simulink model "Mainframe"  (R2021a)
settings: Solver=FixedStepAuto  StartTime=0.0  StopTime=60  FixedStep=0.001  RelTol=1e-3
values from neighbouring files (symbols this model uses):
  den_lpf_d = den_lpf20    [Mainframe_init.m]    (also in load_autopilot.m)
  Emulated_FCC_IO_Delay = 7    [Mainframe_init.m]
  Enable_Gyros = 0    [Mainframe_init.m]
  Enable_INS = 0    [Mainframe_init.m]
  num_lpf_d = num_lpf20    [Mainframe_init.m]    (also in load_autopilot.m)
undefined symbols (not defined in the file or in its folder): act_dmp, act_omega, Actuator, Aerodynamics, aMode, Autopilot, AUX, c_b_WGS, c_be, c_flat, c_grav, c_h_geop0, c_h_geope, c_pa0, c_pe, c_r0, c_rot, c_rsma, c_Tmp0, d_siB_0, d_siB_max, d_siB_min, dd_siB_max, dd_siB_min, dev, DiscIntNeverNeededParam, e_pa, e_Tmp, fin_maxrate, flag_I_act_switch, flag_I_aero_switch, flag_I_flat, flag_I_gravity_switch, flag_I_rot, hcr, HIL_Data, JMMM_0, JMMM_e, JSPB_e, lat_0, lon_0, Mass_Props, mB_0, mM_0, mM_e, National_Instruments, Newton, pBII_0, PCIe, pMPB, pNPB, propellant_kg, prp_FBPB, prp_mdot, prp_T, pSPB, pwm_output1, qEG_0, qIB_0, qIE_0 ... (+31)
libraries: simulink_extras x38, simulink x31, custom_blocks x11, sldrtlib x10, aerolibcommonsys x4, px4Sensorslib x3, px4lib x3, aerolibnav x1
(part 5 of 17)

== system Mainframe/Non-linear Flight Dynamic Model/GRM_Airframe/weight_and_balance/center_of_gravity ==
  mB : Inport
  mM : Inport  Port=2
  1-D Lookup Table : Lookup_n-D  NumberOfTableDimensions=1  BreakpointsForDimension1=Mass_Props.propellant_bkpts  Table=Mass_Props.CGx_m_tbl  ExtrapMethod=Clip  UseLastTableValue=on  InternalRulePriority=Speed  RndMeth=Simplest  InputSameDT=on
      settings: AttributesFormatString=|
      | %<Table>
      | %<BreakpointsForDimension1>
  1-D Lookup Table3 : Lookup_n-D  NumberOfTableDimensions=1  BreakpointsForDimension1=Mass_Props.propellant_bkpts  Table=Mass_Props.CGy_m_tbl  ExtrapMethod=Clip  UseLastTableValue=on  InternalRulePriority=Speed  RndMeth=Simplest  InputSameDT=on
      settings: AttributesFormatString=|
      | %<Table>
      | %<BreakpointsForDimension1>
  1-D Lookup Table6 : Lookup_n-D  NumberOfTableDimensions=1  BreakpointsForDimension1=Mass_Props.propellant_bkpts  Table=Mass_Props.CGz_m_tbl  ExtrapMethod=Clip  UseLastTableValue=on  InternalRulePriority=Speed  RndMeth=Simplest  InputSameDT=on
      settings: AttributesFormatString=|
      | %<Table>
      | %<BreakpointsForDimension1>
  Add6 : Sum
  Add7 : Sum
  Add8 : Sum
  Constant10 : Constant  Value=unc_cg_x
  Constant11 : Constant  Value=unc_cg_y
  Constant12 : Constant  Value=unc_cg_z
  Terminator1 : Terminator
  Vector Concatenate1 : Concatenate  NumInputs=3
  mM D2 : InportShadow  Port=2
  mM D3 : InportShadow  Port=2
  pBPB : Outport  VectorParamsAs1DForOutWhenUnconnected=off
  wires:
  1-D Lookup Table6/1 -> Add8/1
  1-D Lookup Table3/1 -> Add7/1
  Vector Concatenate1/1 -> pBPB/1  "pBPB"
  1-D Lookup Table/1 -> Add6/1
  mM/1 -> 1-D Lookup Table/1
  mM D2/1 -> 1-D Lookup Table3/1
  mM D3/1 -> 1-D Lookup Table6/1
  Add6/1 -> Vector Concatenate1/1
  Constant10/1 -> Add6/2
  Constant11/1 -> Add7/2
  Add7/1 -> Vector Concatenate1/2
  Constant12/1 -> Add8/2
  Add8/1 -> Vector Concatenate1/3
  mB/1 -> Terminator1/1

== system Mainframe/Non-linear Flight Dynamic Model/GRM_Airframe/weight_and_balance/mass ==
  sim_time_launch : Inport
  1-D Lookup Table2 : Lookup_n-D  NumberOfTableDimensions=1  BreakpointsForDimension1=prp_T  Table=prp_mdot  ExtrapMethod=Clip  DiagnosticForOutOfRangeInput=Warning  UseLastTableValue=on  InternalRulePriority=Speed  RndMeth=Simplest  InputSameDT=on
  Constant : Constant  Value=0
  Constant1 : Constant  Value=mB_0
  Constant2 : Constant  Value=propellant_kg
      settings: AttributesFormatString=%<Value>
  Gain : Gain  Gain=-1
  Integrator1 : Integrator  InitialConditionSource=external
  Saturation : Saturate  UpperLimit=prp_T(end)  LowerLimit=0
      settings: AttributesFormatString=|
      | %<UpperLimit>
      | %<LowerLimit>
  Subtract1 : Sum
  Switch : Switch  Criteria=u2 > Threshold
  Switch1 : Switch  Criteria=u2 > Threshold
  mB_c : Outport  VectorParamsAs1DForOutWhenUnconnected=off
  mM : Outport  Port=2  VectorParamsAs1DForOutWhenUnconnected=off
  wires:
  Constant1/1 -> Subtract1/1
  Subtract1/1 -> mB_c/1  "mB_c"
  Switch/1 -> Switch1/2, Switch1/3, Saturation/1
  Constant/1 -> Switch/3
  sim_time_launch/1 -> Switch/1, Switch/2
  Saturation/1 -> 1-D Lookup Table2/1
  Switch1/1 -> mM/1, Subtract1/2  "mM"
  Constant2/1 -> Integrator1/2
  1-D Lookup Table2/1 -> Gain/1  "mdot_kgps"
  Gain/1 -> Integrator1/1
  Integrator1/1 -> Switch1/1  "propellant_remaining_kg"

== system Mainframe/Non-linear Flight Dynamic Model/GRM_Airframe/weight_and_balance/mass_uncertainty ==
  mB_c : Inport
  Add : Sum
  Constant : Constant  Value=unc_mB_bl
  Constant1 : Constant  Value=unc_mB_scale
  Product : Product
  mB : Outport  VectorParamsAs1DForOutWhenUnconnected=off
  wires:
  Constant/1 -> Add/1
  mB_c/1 -> Product/1
  Add/1 -> mB/1  "mB"
  Constant1/1 -> Product/2
  Product/1 -> Add/2

== system Mainframe/Non-linear Flight Dynamic Model/GRM_Airframe/weight_and_balance/moi ==
  pBPB : Inport
  mM : Inport  Port=2
  1-D Lookup Table : Lookup_n-D  NumberOfTableDimensions=1  BreakpointsForDimension1=Mass_Props.propellant_bkpts  Table=Mass_Props.Ixx_tbl  ExtrapMethod=Clip  UseLastTableValue=on  InternalRulePriority=Speed  RndMeth=Simplest  InputSameDT=on
      settings: AttributesFormatString=|
      | %<Table>
      | %<BreakpointsForDimension1>
  1-D Lookup Table1 : Lookup_n-D  NumberOfTableDimensions=1  BreakpointsForDimension1=Mass_Props.propellant_bkpts  Table=Mass_Props.Ixy_tbl  ExtrapMethod=Clip  UseLastTableValue=on  InternalRulePriority=Speed  RndMeth=Simplest  InputSameDT=on
      settings: AttributesFormatString=|
      | %<Table>
      | %<BreakpointsForDimension1>
  1-D Lookup Table2 : Lookup_n-D  NumberOfTableDimensions=1  BreakpointsForDimension1=Mass_Props.propellant_bkpts  Table=Mass_Props.Ixz_tbl  ExtrapMethod=Clip  UseLastTableValue=on  InternalRulePriority=Speed  RndMeth=Simplest  InputSameDT=on
      settings: AttributesFormatString=|
      | %<Table>
      | %<BreakpointsForDimension1>
  1-D Lookup Table3 : Lookup_n-D  NumberOfTableDimensions=1  BreakpointsForDimension1=Mass_Props.propellant_bkpts  Table=Mass_Props.Iyx_tbl  ExtrapMethod=Clip  UseLastTableValue=on  InternalRulePriority=Speed  RndMeth=Simplest  InputSameDT=on
      settings: AttributesFormatString=|
      | %<Table>
      | %<BreakpointsForDimension1>
  1-D Lookup Table4 : Lookup_n-D  NumberOfTableDimensions=1  BreakpointsForDimension1=Mass_Props.propellant_bkpts  Table=Mass_Props.Iyy_tbl  ExtrapMethod=Clip  UseLastTableValue=on  InternalRulePriority=Speed  RndMeth=Simplest  InputSameDT=on
      settings: AttributesFormatString=|
      | %<Table>
      | %<BreakpointsForDimension1>
  1-D Lookup Table5 : Lookup_n-D  NumberOfTableDimensions=1  BreakpointsForDimension1=Mass_Props.propellant_bkpts  Table=Mass_Props.Iyz_tbl  ExtrapMethod=Clip  UseLastTableValue=on  InternalRulePriority=Speed  RndMeth=Simplest  InputSameDT=on
      settings: AttributesFormatString=|
      | %<Table>
      | %<BreakpointsForDimension1>
  1-D Lookup Table6 : Lookup_n-D  NumberOfTableDimensions=1  BreakpointsForDimension1=Mass_Props.propellant_bkpts  Table=Mass_Props.Izx_tbl  ExtrapMethod=Clip  UseLastTableValue=on  InternalRulePriority=Speed  RndMeth=Simplest  InputSameDT=on
      settings: AttributesFormatString=|
      | %<Table>
      | %<BreakpointsForDimension1>
  1-D Lookup Table7 : Lookup_n-D  NumberOfTableDimensions=1  BreakpointsForDimension1=Mass_Props.propellant_bkpts  Table=Mass_Props.Izy_tbl  ExtrapMethod=Clip  UseLastTableValue=on  InternalRulePriority=Speed  RndMeth=Simplest  InputSameDT=on
      settings: AttributesFormatString=|
      | %<Table>
      | %<BreakpointsForDimension1>
  1-D Lookup Table8 : Lookup_n-D  NumberOfTableDimensions=1  BreakpointsForDimension1=Mass_Props.propellant_bkpts  Table=Mass_Props.Izz_tbl  ExtrapMethod=Clip  UseLastTableValue=on  InternalRulePriority=Speed  RndMeth=Simplest  InputSameDT=on
      settings: AttributesFormatString=|
      | %<Table>
      | %<BreakpointsForDimension1>
  Add : Sum  Commented=on
  Add4 : Sum  Commented=on
  Add5 : Sum  Commented=on
  Constant15 : Constant  Commented=on  Value=JSPB_e
  JMMM_linear_interpolation : Subsystem  Commented=on
  Matrix Concatenate : Concatenate  NumInputs=3  Mode=Multidimensional array  ConcatenateDimension=2
  Terminator : Terminator  Commented=on
  Vector Concatenate : Concatenate  NumInputs=3
  Vector Concatenate1 : Concatenate  NumInputs=3
  Vector Concatenate2 : Concatenate  NumInputs=3
  mM D{1..9} (9 alike) : InportShadow  Port=2
  moi_coordinate_transformation : Subsystem  Commented=on
  moi_uncertainty : Subsystem
  steiners_theorem_missile : Subsystem  Commented=on
  steiners_theorem_motor : Subsystem  Commented=on
  JBBB : Outport  VectorParamsAs1DForOutWhenUnconnected=off
  wires:
  mM/1 -> steiners_theorem_motor/2(mM), JMMM_linear_interpolation/1(mM)
  JMMM_linear_interpolation/1(JMMM) -> moi_coordinate_transformation/1(JMMM)
  moi_coordinate_transformation/1(JMMB) -> Add/2
  pBPB/1 -> steiners_theorem_missile/1(pBPB), steiners_theorem_motor/1(pBPB)
  steiners_theorem_motor/1(JM_deviation) -> Add/1
  Add/1 -> Add4/2  "JMBB"
  Constant15/1 -> Add5/1
  Add5/1 -> Add4/1  "JSBB"
  steiners_theorem_missile/1(J_deviation) -> Add5/2
  Add4/1 -> Terminator/1  "JBBB_c"
  moi_uncertainty/1(JBBB) -> JBBB/1
  mM D1/1 -> 1-D Lookup Table/1
  mM D2/1 -> 1-D Lookup Table3/1
  mM D3/1 -> 1-D Lookup Table6/1
  mM D4/1 -> 1-D Lookup Table1/1
  mM D5/1 -> 1-D Lookup Table4/1
  mM D6/1 -> 1-D Lookup Table7/1
  mM D7/1 -> 1-D Lookup Table2/1
  mM D8/1 -> 1-D Lookup Table5/1
  mM D9/1 -> 1-D Lookup Table8/1
  1-D Lookup Table6/1 -> Vector Concatenate/3
  1-D Lookup Table3/1 -> Vector Concatenate/2
  1-D Lookup Table/1 -> Vector Concatenate/1
  1-D Lookup Table1/1 -> Vector Concatenate1/1
  1-D Lookup Table4/1 -> Vector Concatenate1/2
  1-D Lookup Table7/1 -> Vector Concatenate1/3
  1-D Lookup Table2/1 -> Vector Concatenate2/1
  1-D Lookup Table5/1 -> Vector Concatenate2/2
  1-D Lookup Table8/1 -> Vector Concatenate2/3
  Vector Concatenate/1 -> [MOI_matrix_col1]
  Vector Concatenate1/1 -> [MOI_matrix_col2]
  Vector Concatenate2/1 -> [MOI_matrix_col3]
  [MOI_matrix_col1] -> Matrix Concatenate/1
  [MOI_matrix_col2] -> Matrix Concatenate/2
  [MOI_matrix_col3] -> Matrix Concatenate/3
  Matrix Concatenate/1 -> moi_uncertainty/1(JBBB_c)  "JBBB_c"

== system Mainframe/Non-linear Flight Dynamic Model/Subsystem1/Extract States/Assemble_States_Bus1 ==
  Translation_States : Inport
  Rotation_States : Inport  Port=2
  Translation_States_Dot : Inport  Port=3
  Rotation_States_Dot : Inport  Port=4
  Attitude_States : Inport  Port=5
  POS_NED : Inport  Port=6
  POS_NED_dot : Inport  Port=7
  Bus Creator{1,4..6,8,12..13} (7 alike) : BusCreator  Inputs=3
  Bus Creator3 : BusCreator  Inputs=7
  Bus Creator7 : BusCreator  Inputs=2
  Bus Creator9 : BusCreator  Inputs=4
  Demux : Demux
  Demux{1..7} (7 alike) : Demux  Outputs=3
  Rotation Angles to Quaternions : Subsystem  mask(Ang2Quat){rotationOrder=ZYX, aMode=aMode}
      mask prompts: rotationOrder "shared_aeroblks:sharedaeroblktransform:blockAng2QuatParamRotationOrder"
      mask help: shared_aeroblks:sharedaeroblktransform:blockAng2QuatDesc
      mask init:
      | if aerosharedtest(gcb)
      |     ports=aerosharedicon('sharedang2quat');
      | else
      |     ports=sharedautoicon('sharedang2quat');
      | end
      settings: AttributesFormatString=Rotation Order: %<rotationOrder>
      mask Help: eval('if license(''test'',''Aerospace_Blockset'')aerosharedhelp(''rotation_angles_to_quaternions'');elseif license(''test'',''Powertrain_Blockset'')sharedautohelp(''rotation_angles_to_quaternions'');end')
      mask TypeOptions rotationOrder: shared_aeroblks:sharedaeroblktransform:blockParamComboZYX | shared_aeroblks:sharedaeroblktransform:blockParamComboZYZ | shared_aeroblks:sharedaeroblktransform:blockParamComboZXY | shared_aeroblks:sharedaeroblktransform:blockParamComboZXZ | shared_aeroblks:sharedaeroblktransform:blockParamComboYXZ | shared_aeroblks:sharedaeroblktransform:blockParamComboYXY | shared_aeroblks:sharedaeroblktransform:blockParamComboYZX | shared_aeroblks:sharedaeroblktransform:blockParamComboYZY | shared_aeroblks:sharedaeroblktransform:blockParamComboXYZ | shared_aeroblks:sharedaeroblktransform:blockParamComboXYX | shared_aeroblks:sharedaeroblktransform:blockParamComboXZY | shared_aeroblks:sharedaeroblktransform:blockParamComboXZX
      mask DialogControl rotationOrder Prompt: Rotation order:
      mask Display:
      | port_label('input',1,'[R_1,R_2,R_3]','texmode','on')
      | port_label('output',1,'q','texmode','on')
  Selector : Selector  InputPortWidth=3  IndexOptions=Index vector (dialog)  Indices=[3,2,1]  OutputSizes=1
  Three-axis Inertial Measurement Unit3 : Subsystem  Commented=on  mask(Three-axis Inertial Measurement Unit){units=Metric (MKS), imu=[0 0 0], i_Ts=0, dtype_a=on, w_a=190, z_a=0.707, a_sf_cc=[1 0 0; 0 1 0; 0 0 1], a_bias=[0 0 0], a_sat=[-inf  -inf  -inf  inf inf inf], dtype_g=on, w_g=190, z_g=0.707, g_sf_cc=[1 0 0; 0 1 0; 0 0 1], g_bias=[0 0 0], g_sens=[0 0 0], g_sat=[-inf  -inf  -inf  inf inf inf], i_rand=on, i_seeds=[23093 23094 23095 23096 23097 23098], i_pow=[0.001 0.001 0.001 0.0001 0.0001 0.0001]}
      mask prompts: units "aeroblks:aeroblknav:blockThreeaxisInertialMeasurementUnitParamUnits"; imu "aeroblks:aeroblknav:blockThreeaxisInertialMeasurementUnitParamIMUlocation"; i_Ts "aeroblks:aeroblknav:blockThreeaxisInertialMeasurementUnitParamUpdaterate"; dtype_a "aeroblks:aeroblknav:blockThreeaxisInertialMeasurementUnitParamSecondorderdynamicsforaccelerometer"; w_a "aeroblks:aeroblknav:blockThreeaxisInertialMeasurementUnitParamAccelerometernaturalfrequencyradsec"; z_a "aeroblks:aeroblknav:blockThreeaxisInertialMeasurementUnitParamAccelerometerdampingratio"; a_sf_cc "aeroblks:aeroblknav:blockThreeaxisInertialMeasurementUnitParamAccelerometerscalefactorandcrosscoupling"; a_bias "aeroblks:aeroblknav:blockThreeaxisInertialMeasurementUnitParamAccelerometermeasurementbias"; a_sat "aeroblks:aeroblknav:blockThreeaxisInertialMeasurementUnitParamAccelerometerupperandlowerlimits"; dtype_g "aeroblks:aeroblknav:blockThreeaxisInertialMeasurementUnitParamSecondorderdynamicsforgyro"; w_g "aeroblks:aeroblknav:blockThreeaxisInertialMeasurementUnitParamGyronaturalfrequencyradsec"; z_g "aeroblks:aeroblknav:blockThreeaxisInertialMeasurementUnitParamGyrodampingratio"; g_sf_cc "aeroblks:aeroblknav:blockThreeaxisInertialMeasurementUnitParamGyroscalefactorsandcrosscoupling"; g_bias "aeroblks:aeroblknav:blockThreeaxisInertialMeasurementUnitParamGyromeasurementbias"; g_sens "aeroblks:aeroblknav:blockThreeaxisInertialMeasurementUnitParamGsensitivebias"; g_sat "aeroblks:aeroblknav:blockThreeaxisInertialMeasurementUnitParamGyroupperandlowerlimits"; i_rand "aeroblks:aeroblknav:blockThreeaxisInertialMeasurementUnitParamNoiseon"; i_seeds "aeroblks:aeroblknav:blockThreeaxisInertialMeasurementUnitParamNoiseseeds"; i_pow "aeroblks:aeroblknav:blockThreeaxisInertialMeasurementUnitParamNoisepower"
      mask help: aeroblks:aeroblknav:blockThreeaxisInertialMeasurementUnitDesc
      mask init:
      | block = gcb;   
      | ports=aeroicon('aeroblkimu','icon');
      mask Help: eval('asbhelp');
      mask TypeOptions units: aeroblks:aeroblknav:blockThreeaxisInertialMeasurementUnitParamComboMetricMKS | aeroblks:aeroblknav:blockThreeaxisInertialMeasurementUnitParamComboEnglish
      mask Callback dtype_a: aeroicon('aeroblkimu')
      mask Callback dtype_g: aeroicon('aeroblkimu')
      mask Callback i_rand: aeroicon('aeroblkimu')
      mask DialogControl ParameterTabVar0 Prompt: Main
      mask DialogControl units Prompt: Units:
      mask DialogControl imu Prompt: IMU location:
      mask DialogControl i_Ts Prompt: Update rate:
      mask DialogControl ParameterTabVar01 Prompt: Accelerometer
      mask DialogControl dtype_a Prompt: Second-order dynamics for accelerometer
      mask DialogControl w_a Prompt: Accelerometer natural frequency (rad/sec):
      mask DialogControl z_a Prompt: Accelerometer damping ratio:
      mask DialogControl a_sf_cc Prompt: Accelerometer scale factor and cross-coupling:
      mask DialogControl a_bias Prompt: Accelerometer measurement bias:
      mask DialogControl a_sat Prompt: Accelerometer upper and lower limits:
      mask DialogControl ParameterTabVar012 Prompt: Gyroscope
      mask DialogControl dtype_g Prompt: Second-order dynamics for gyro
      mask DialogControl w_g Prompt: Gyro natural frequency (rad/sec):
      mask DialogControl z_g Prompt: Gyro damping ratio:
      mask DialogControl g_sf_cc Prompt: Gyro scale factors and cross-coupling:
      mask DialogControl g_bias Prompt: Gyro measurement bias:
      mask DialogControl g_sens Prompt: G-sensitive bias:
      mask DialogControl g_sat Prompt: Gyro upper and lower limits:
      mask DialogControl ParameterTabVar0123 Prompt: Noise
      mask DialogControl i_rand Prompt: Noise on
      mask DialogControl i_seeds Prompt: Noise seeds:
      mask DialogControl i_pow Prompt: Noise power:
      mask Display:
      | port_label(ports(1).type,ports(1).port,ports(1).txt,'texmode','on');
      | port_label(ports(2).type,ports(2).port,ports(2).txt,'texmode','on');
      | port_label(ports(3).type,ports(3).port,ports(3).txt,'texmode','on');
      | port_label(ports(4).type,ports(4).port,ports(4).txt,'texmode','on');
      | port_label(ports(5).type,ports(5).port,ports(5).txt,'texmode','on');
      | port_label(ports(6).type,ports(6).port,ports(6).txt,'texmode','on');
      | port_label(ports(7).type,ports(7).port,ports(7).txt,'texmode','on');
  States : Outport  VectorParamsAs1DForOutWhenUnconnected=off
  wires:
  Bus Creator7/1 -> Bus Creator3/5  "Attitude_States"
  Demux/3 -> Bus Creator9/3  "quat_2"
  Demux/4 -> Bus Creator9/4  "quat_3"
  Demux/1 -> Bus Creator9/1  "quat_0"
  Bus Creator9/1 -> Bus Creator7/2  "ATT_Quaternions"
  Bus Creator12/1 -> Bus Creator3/6  "POS_NED"
  Demux/2 -> Bus Creator9/2  "quat_1"
  Bus Creator8/1 -> Bus Creator7/1  "ATT_Euler"
  Bus Creator4/1 -> Bus Creator3/1  "Translation_States"
  Bus Creator6/1 -> Bus Creator3/2  "Rotation_States"
  Bus Creator5/1 -> Bus Creator3/3  "Translation_States_Dot"
  Rotation Angles to Quaternions/1(Quat) -> Demux/1
  Demux6/3 -> Bus Creator12/3  "POS_z_NED_m"
  Demux6/2 -> Bus Creator12/2  "POS_y_NED_m"
  Demux6/1 -> Bus Creator12/1  "POS_x_NED_m"
  Demux5/3 -> Bus Creator8/3  "Psi_rad"
  Demux5/2 -> Bus Creator8/2  "Theta_rad"
  Demux5/1 -> Bus Creator8/1  "Phi_rad"
  Demux2/3 -> Bus Creator6/3  "r_radDs"
  Demux2/2 -> Bus Creator6/2  "q_radDs"
  Demux2/1 -> Bus Creator6/1  "p_radDs"
  Demux3/3 -> Bus Creator5/3  "w_dot_mDs2"
  Demux3/2 -> Bus Creator5/2  "v_dot_mDs2"
  Demux3/1 -> Bus Creator5/1  "u_dot_mDs2"
  Demux1/3 -> Bus Creator4/3  "w_mDs"
  Demux1/2 -> Bus Creator4/2  "v_mDs"
  Demux1/1 -> Bus Creator4/1  "u_mDs"
  Bus Creator13/1 -> Bus Creator3/4  "Rotation_States_Dot"
  Demux4/1 -> Bus Creator13/1  "p_dot_radDs2"
  Demux4/2 -> Bus Creator13/2  "q_dot_radDs2"
  Demux4/3 -> Bus Creator13/3  "r_dot_radDs2"
  Translation_States/1 -> Demux1/1
  Rotation_States/1 -> Demux2/1
  Translation_States_Dot/1 -> Demux3/1
  Rotation_States_Dot/1 -> Demux4/1
  Attitude_States/1 -> Selector/1, Demux5/1
  POS_NED/1 -> Demux6/1
  Bus Creator3/1 -> States/1  "FDM_States"
  Selector/1 -> Rotation Angles to Quaternions/1("R1, R2, R3")
  POS_NED_dot/1 -> Demux7/1
  Demux7/2 -> Bus Creator1/2  "POS_y_NED_dot_m"
  Demux7/3 -> Bus Creator1/3  "POS_z_NED_dot_m"
  Bus Creator1/1 -> Bus Creator3/7  "POS_NED_dot"
  Demux7/1 -> Bus Creator1/1  "POS_x_NED_dot_m"

== system Mainframe/Non-linear Flight Dynamic Model/Subsystem1/Extract States/quaternion_to_euler_angles1 ==
  note: Um numerische Probleme zu
      | vermeiden, wird hier eine Saturiierung
      | benutzt.
  note: Outputs [size]:
      |
      | roll angle [1]
      | pitch angle [1]
      | yaw angle [1]
  note: Inputs [size]:
      |
      | quaternion [4]
  q : Inport  PortDimensions=4
  Add : Sum
  Add1 : Sum  Inputs=+--
  Add2 : Sum  Inputs=+-
  Add3 : Sum
  Add4 : Sum  Inputs=+--
  Complex to Real-Imag : ComplexToRealImag  Output=Real
  Constant : Constant  Value=0.5
  Constant1 : Constant  Value=0.5
  Demux : Demux
  Gain : Gain  Gain=2
  Product{,1..9} (10 alike) : Product
  Saturation : Saturate  UpperLimit=1  LowerLimit=-1
      settings: AttributesFormatString=|
      | %<UpperLimit>
      | %<LowerLimit>
  Trigonometric Function : Trigonometry  Operator=atan2
  Trigonometric Function1 : Trigonometry  Operator=asin
  Trigonometric Function2 : Trigonometry  Operator=atan2
  Vector Concatenate : Concatenate  NumInputs=3
  eulx : Outport  VectorParamsAs1DForOutWhenUnconnected=off
  wires:
  Vector Concatenate/1 -> Complex to Real-Imag/1
  Complex to Real-Imag/1 -> eulx/1
  Trigonometric Function2/1 -> Vector Concatenate/3
  Trigonometric Function1/1 -> Vector Concatenate/2
  Trigonometric Function/1 -> Vector Concatenate/1
  Add/1 -> Trigonometric Function/1
  Product1/1 -> Add/2
  Product/1 -> Add/1
  Product3/1 -> Add1/3
  Product2/1 -> Add1/2
  Product5/1 -> Add2/2
  Product4/1 -> Add2/1
  Product7/1 -> Add3/2
  Product6/1 -> Add3/1
  Add3/1 -> Trigonometric Function2/1
  Add4/1 -> Trigonometric Function2/2
  Add2/1 -> Gain/1
  Add1/1 -> Trigonometric Function/2
  q/1 -> Demux/1
  Demux/4 -> Product7/2, Product4/2, Product/2  "4"
  Demux/1 -> Product2/2, Product2/1, Product/1, Product6/1, Product5/1  "1"
  Demux/2 -> Product4/1, Product3/2, Product3/1, Product1/1, Product8/2, Product8/1, Product6/2  "2"
  Constant/1 -> Add1/1
  Product9/1 -> Add4/3
  Product8/1 -> Add4/2
  Constant1/1 -> Add4/1
  Demux/3 -> Product9/2, Product9/1, Product7/1, Product1/2, Product5/2  "3"
  Gain/1 -> Saturation/1
  Saturation/1 -> Trigonometric Function1/1

== system Mainframe/Non-linear Flight Dynamic Model/Subsystem1/Fin Deflections/Degrees to Radians ==
  Degrees in : Inport
  Gain1 : Gain  Gain=pi/180  SaturateOnIntegerOverflow=on  OutDataTypeStr=Inherit: Same as input  ParamDataTypeStr=Inherit: Same as input
  Radians out : Outport  InitialOutput=0  VectorParamsAs1DForOutWhenUnconnected=off
  wires:
  Gain1/1 -> Radians out/1
  Degrees in/1 -> Gain1/1

== system Mainframe/Non-linear Flight Dynamic Model/Subsystem1/Fin Deflections/Degrees to Radians1 ==
  Degrees in : Inport
  Gain1 : Gain  Gain=pi/180  SaturateOnIntegerOverflow=on  OutDataTypeStr=Inherit: Same as input  ParamDataTypeStr=Inherit: Same as input
  Radians out : Outport  InitialOutput=0  VectorParamsAs1DForOutWhenUnconnected=off
  wires:
  Gain1/1 -> Radians out/1
  Degrees in/1 -> Gain1/1

== system Mainframe/Non-linear Flight Dynamic Model/Subsystem1/Fin Deflections/Degrees to Radians2 ==
  Degrees in : Inport
  Gain1 : Gain  Gain=pi/180  SaturateOnIntegerOverflow=on  OutDataTypeStr=Inherit: Same as input  ParamDataTypeStr=Inherit: Same as input
  Radians out : Outport  InitialOutput=0  VectorParamsAs1DForOutWhenUnconnected=off
  wires:
  Gain1/1 -> Radians out/1
  Degrees in/1 -> Gain1/1

== system Mainframe/Non-linear Flight Dynamic Model/Subsystem1/Fin Deflections/control_allocation ==
  fin_cmd : Inport
  Constant7 : Constant  Value=Tr4r3
  Product : Product  Multiplication=Matrix(*)
  siB_cmd : Outport  VectorParamsAs1DForOutWhenUnconnected=off
  wires:
  Product/1 -> siB_cmd/1  "siB_cmd"
  fin_cmd/1 -> Product/2
  Constant7/1 -> Product/1

== system Mainframe/Non-linear Flight Dynamic Model/Subsystem1/GRM_Airframe/aerodynamics ==
  str_flow : Inport
  fin : Inport  Port=2
  wab : Inport  Port=3
  env_glbl : Inport  Port=4
  Bus Selector : BusSelector  OutputSignals=qdynB,MaB,alB,beB,hBE,wBIB_star
  Bus Selector1 : BusSelector  OutputSignals=afinB
  Bus Selector2 : BusSelector  OutputSignals=pBPB
  aerodynamic_via_lookup : Subsystem
  logic_base_drag : Subsystem
  aero : Outport  VectorParamsAs1DForOutWhenUnconnected=off
  wires:
  str_flow/1 -> Bus Selector/1
  wab/1 -> Bus Selector2/1
  fin/1 -> Bus Selector1/1
  Bus Selector2/1 -> aerodynamic_via_lookup/1(pBPB)  "<pBPB>"
  Bus Selector/1 -> aerodynamic_via_lookup/2(qdynB)  "<qdynB>"
  Bus Selector/2 -> aerodynamic_via_lookup/3(MaB)  "<MaB>"
  Bus Selector/3 -> aerodynamic_via_lookup/4(alB)  "<alB>"
  Bus Selector/4 -> aerodynamic_via_lookup/5(beB)  "<beB>"
  Bus Selector/5 -> aerodynamic_via_lookup/6(hBE)  "<hBE>"
  Bus Selector1/1 -> aerodynamic_via_lookup/8(afinB)  "<afinB>"
  Bus Selector/6 -> aerodynamic_via_lookup/7(wBIB_star)  "<wBIB_star>"
  aerodynamic_via_lookup/1(aero_bus) -> aero/1
  env_glbl/1 -> logic_base_drag/1(env_glbl)
  logic_base_drag/1(flag_base_drag) -> aerodynamic_via_lookup/9(flag_I_prp)

== system Mainframe/Non-linear Flight Dynamic Model/Subsystem1/GRM_Airframe/environment ==
  flight_dyn : Inport
  env_glbl : Inport  Port=2
  Bus Creator1 : BusCreator  Inputs=2
  Bus Creator2 : BusCreator  Inputs=2
  Bus Selector : BusSelector  OutputSignals=lon,lat,hBE
  Bus Selector1 : BusSelector  OutputSignals=atm_dyn_bus
  Saturation : Saturate  UpperLimit=inf  LowerLimit=eps
      settings: AttributesFormatString=|
      | %<UpperLimit>
      | %<LowerLimit>
  WGS84_Gravitation : Subsystem  mask{flg_omega_enabled=on}
      mask prompts: flg_omega_enabled "Zentripetalbeschleunigung mitberechnen"
      mask help:
      | Dieser Block berechnet die Gravitation für das idealisierte WGS84
      | Ellipsoid. Die Berechnung ist hierbei nach dem Technical Report
      | "Department of Defense World Geodetic System 1984", NIMA TR8350.2,
      | Third Edition, Amendment 1 vom 3 Januar 2000 implementiert.
      | Das Modell ist gültig für alle Höhen über dem WGS84 Referenzellipsoid, und
      | ist somit der reinen Taylorexpansion des Somigliana Modells überlegen
      | (siehe Kapitel 4.3 des WGS84 reports).
      |
      | ---------------------------------------------------------------------------
      | Longitude [rad]: Nach WGS84 definierte Geodätische Länge.  (lambda)
      | Lattitude [rad]: Nach WGS84 definierte Geodätische Breite. (phi)
      | Height [m]: Höhe über dem WGS84 Referenzellipsoid.
      mask init:
      | [ c_rsma, c_b_WGS, c_grav, c_rot] = init_WGS84_Gravitationsmodell();
  atmosphere_static_ISO_2533 : Subsystem
  convert_to_local_frame : Subsystem
  env : Outport  VectorParamsAs1DForOutWhenUnconnected=off
  wires:
  convert_to_local_frame/1(gBG) -> Bus Creator2/1
  flight_dyn/1 -> Bus Selector/1
  WGS84_Gravitation/1(gE) -> convert_to_local_frame/1(gE)
  Bus Selector/1 -> WGS84_Gravitation/1(lon)  "<lon>"
  Bus Selector/3 -> atmosphere_static_ISO_2533/1(hBE), Saturation/1  "<hBE>"
  Bus Creator2/1 -> env/1  "env_bus"
  Bus Selector/2 -> WGS84_Gravitation/2(lat)  "<lat>"
  Bus Creator1/1 -> Bus Creator2/2  "atm_bus"
  Saturation/1 -> WGS84_Gravitation/3(h)
  atmosphere_static_ISO_2533/1(atm_stat) -> Bus Creator1/1  "atm_stat_bus"
  env_glbl/1 -> Bus Selector1/1, atmosphere_static_ISO_2533/2(env_glbl)
  Bus Selector1/1 -> Bus Creator1/2  "<atm_dyn_bus>"

== system Mainframe/Non-linear Flight Dynamic Model/Subsystem1/GRM_Airframe/fin_actuators ==
  cmd : Inport
  Bus Creator3 : BusCreator  Inputs=7
  Bus Selector : BusSelector  OutputSignals=siB_cmd
  Constant : Constant  Value=flag_I_act_switch
  Constant7 : Constant  Value=tRRR
  Demux : Demux
  Rudder : Subsystem  mask{siB_max=siB_max, siB_min=siB_min, d_siB_max=d_siB_max, d_siB_min=d_siB_min, dd_siB_max=dd_siB_max, dd_siB_min=dd_siB_min, omega=act_omega, dmp=act_dmp, unc_bl=unc_act_bl, unc_scale=unc_act_scale, unc_off=unc_act_off, siB_0=siB_0, d_siB_0=d_siB_0}
      mask prompts: siB_max "Obere Limitierung des Ruderstellwinkels in [rad]"; siB_min "Untere Limitierung des Ruderstellwinkels in [rad]"; d_siB_max "Obere Limitierung der Ruderstellwinkelgeschwindigkeit in [rad/s]"; d_siB_min "Untere Limitierung der Ruderstellwinkelgeschwindigkeit in [rad/s]"; dd_siB_max "Obere Limitierung der Ruderstellwinkelbeschleunigung in [rad/s^2]"; dd_siB_min "Untere Limitierung der Ruderstellwinkelbeschleunigung in [rad/s^2]"; omega "Eckfrequenz in [Hz]"; dmp "Dämpfung in [kg/s]"; unc_bl "Rückschlag des Aktuators (Backlash) in [rad]"; unc_scale "Skalenfehler in [-]"; unc_off "Versatz (Offset) in [rad]"; siB_0 "Startwert Ruderwinkel in [rad]"; d_siB_0 "Startwert Ruderwinkelgeschwindigkeiten in [rad/s]"
      mask DialogControl ParameterGroupVar Prompt: Limitierungen
      mask DialogControl Container3 Prompt: Dynamik
      mask DialogControl Container4 Prompt: Aktuatorfehler
      mask DialogControl Container5 Prompt: Startwerte
  Rudder1 : Subsystem  mask{siB_max=siB_max, siB_min=siB_min, d_siB_max=d_siB_max, d_siB_min=d_siB_min, dd_siB_max=dd_siB_max, dd_siB_min=dd_siB_min, omega=act_omega, dmp=act_dmp, unc_bl=unc_act_bl, unc_scale=unc_act_scale, unc_off=unc_act_off, siB_0=siB_0, d_siB_0=d_siB_0}
      mask prompts: siB_max "Obere Limitierung des Ruderstellwinkels in [rad]"; siB_min "Untere Limitierung des Ruderstellwinkels in [rad]"; d_siB_max "Obere Limitierung der Ruderstellwinkelgeschwindigkeit in [rad/s]"; d_siB_min "Untere Limitierung der Ruderstellwinkelgeschwindigkeit in [rad/s]"; dd_siB_max "Obere Limitierung der Ruderstellwinkelbeschleunigung in [rad/s^2]"; dd_siB_min "Untere Limitierung der Ruderstellwinkelbeschleunigung in [rad/s^2]"; omega "Eckfrequenz in [Hz]"; dmp "Dämpfung in [kg/s]"; unc_bl "Rückschlag des Aktuators (Backlash) in [rad]"; unc_scale "Skalenfehler in [-]"; unc_off "Versatz (Offset) in [rad]"; siB_0 "Startwert Ruderwinkel in [rad]"; d_siB_0 "Startwert Ruderwinkelgeschwindigkeiten in [rad/s]"
      mask DialogControl ParameterGroupVar Prompt: Limitierungen
      mask DialogControl Container3 Prompt: Dynamik
      mask DialogControl Container4 Prompt: Aktuatorfehler
      mask DialogControl Container5 Prompt: Startwerte
  Rudder2 : Subsystem  mask{siB_max=siB_max, siB_min=siB_min, d_siB_max=d_siB_max, d_siB_min=d_siB_min, dd_siB_max=dd_siB_max, dd_siB_min=dd_siB_min, omega=act_omega, dmp=act_dmp, unc_bl=unc_act_bl, unc_scale=unc_act_scale, unc_off=unc_act_off, siB_0=siB_0, d_siB_0=d_siB_0}
      mask prompts: siB_max "Obere Limitierung des Ruderstellwinkels in [rad]"; siB_min "Untere Limitierung des Ruderstellwinkels in [rad]"; d_siB_max "Obere Limitierung der Ruderstellwinkelgeschwindigkeit in [rad/s]"; d_siB_min "Untere Limitierung der Ruderstellwinkelgeschwindigkeit in [rad/s]"; dd_siB_max "Obere Limitierung der Ruderstellwinkelbeschleunigung in [rad/s^2]"; dd_siB_min "Untere Limitierung der Ruderstellwinkelbeschleunigung in [rad/s^2]"; omega "Eckfrequenz in [Hz]"; dmp "Dämpfung in [kg/s]"; unc_bl "Rückschlag des Aktuators (Backlash) in [rad]"; unc_scale "Skalenfehler in [-]"; unc_off "Versatz (Offset) in [rad]"; siB_0 "Startwert Ruderwinkel in [rad]"; d_siB_0 "Startwert Ruderwinkelgeschwindigkeiten in [rad/s]"
      mask DialogControl ParameterGroupVar Prompt: Limitierungen
      mask DialogControl Container3 Prompt: Dynamik
      mask DialogControl Container4 Prompt: Aktuatorfehler
      mask DialogControl Container5 Prompt: Startwerte
  Rudder3 : Subsystem  mask{siB_max=siB_max, siB_min=siB_min, d_siB_max=d_siB_max, d_siB_min=d_siB_min, dd_siB_max=dd_siB_max, dd_siB_min=dd_siB_min, omega=act_omega, dmp=act_dmp, unc_bl=unc_act_bl, unc_scale=unc_act_scale, unc_off=unc_act_off, siB_0=siB_0, d_siB_0=d_siB_0}
      mask prompts: siB_max "Obere Limitierung des Ruderstellwinkels in [rad]"; siB_min "Untere Limitierung des Ruderstellwinkels in [rad]"; d_siB_max "Obere Limitierung der Ruderstellwinkelgeschwindigkeit in [rad/s]"; d_siB_min "Untere Limitierung der Ruderstellwinkelgeschwindigkeit in [rad/s]"; dd_siB_max "Obere Limitierung der Ruderstellwinkelbeschleunigung in [rad/s^2]"; dd_siB_min "Untere Limitierung der Ruderstellwinkelbeschleunigung in [rad/s^2]"; omega "Eckfrequenz in [Hz]"; dmp "Dämpfung in [kg/s]"; unc_bl "Rückschlag des Aktuators (Backlash) in [rad]"; unc_scale "Skalenfehler in [-]"; unc_off "Versatz (Offset) in [rad]"; siB_0 "Startwert Ruderwinkel in [rad]"; d_siB_0 "Startwert Ruderwinkelgeschwindigkeiten in [rad/s]"
      mask DialogControl ParameterGroupVar Prompt: Limitierungen
      mask DialogControl Container3 Prompt: Dynamik
      mask DialogControl Container4 Prompt: Aktuatorfehler
      mask DialogControl Container5 Prompt: Startwerte
  Switch : Switch  Criteria=u2 > Threshold
  Vector Concatenate1 : Concatenate  NumInputs=4
  Vector Concatenate2 : Concatenate  NumInputs=4
  Vector Concatenate3 : Concatenate  NumInputs=4
  control_allocation : Subsystem
  fin : Outport  VectorParamsAs1DForOutWhenUnconnected=off
  wires:
  [d_siB3] -> Vector Concatenate2/3
  Demux/4 -> Rudder3/1(siB_c)
  Rudder2/2(d_siB) -> [d_siB3]
  Rudder3/1(siB) -> Vector Concatenate1/4
  Rudder1/2(d_siB) -> [d_siB2]
  Rudder2/1(siB) -> Vector Concatenate1/3
  [d_siB4] -> Vector Concatenate2/4
  [d_siB1] -> Vector Concatenate2/1
  Bus Selector/1 -> Switch/3, Demux/1  "<siB_cmd>"
  [d_siB2] -> Vector Concatenate2/2
  Constant7/1 -> Rudder1/2(tRRR), Rudder3/2(tRRR), Rudder2/2(tRRR), Rudder/2(tRRR)
  [dd_siB2] -> Vector Concatenate3/2
  Demux/3 -> Rudder2/1(siB_c)
  Rudder3/2(d_siB) -> [d_siB4]
  Demux/1 -> Rudder/1(siB_c)
  [dd_siB4] -> Vector Concatenate3/4
  [dd_siB3] -> Vector Concatenate3/3
  cmd/1 -> Bus Selector/1
  [dd_siB1] -> Vector Concatenate3/1
  Rudder1/1(siB) -> Vector Concatenate1/2
  Rudder1/3(dd_siB) -> [dd_siB2]
  Rudder3/3(dd_siB) -> [dd_siB4]
  Rudder/2(d_siB) -> [d_siB1]
  Rudder2/3(dd_siB) -> [dd_siB3]
  Demux/2 -> Rudder1/1(siB_c)
  Rudder/3(dd_siB) -> [dd_siB1]
  Rudder/1(siB) -> Vector Concatenate1/1
  Bus Creator3/1 -> fin/1  "fin_bus"
  Switch/1 -> Bus Creator3/1, control_allocation/1(siB)  "siB"
  Vector Concatenate2/1 -> control_allocation/2(d_siB), Bus Creator3/7  "d_siB"
  Vector Concatenate3/1 -> Bus Creator3/6, control_allocation/3(dd_siB)  "dd_siB"
  control_allocation/1(Tr3r4) -> Bus Creator3/2
  control_allocation/2(finB) -> Bus Creator3/3
  control_allocation/3(d_finB) -> Bus Creator3/4
  control_allocation/4(dd_finB) -> Bus Creator3/5
  Vector Concatenate1/1 -> Switch/1  "siB"
  Constant/1 -> Switch/2

== system Mainframe/Non-linear Flight Dynamic Model/Subsystem1/GRM_Airframe/forces_moments ==
  aero : Inport
  motion_kin : Inport  Port=2
  grav : Inport  Port=3
  prp : Inport  Port=4
  Add : Sum  Inputs=+++
  Add1 : Sum
  Bus Creator : BusCreator  Inputs=2
  Bus Selector : BusSelector  OutputSignals=FBAB,MBAB
  Bus Selector1 : BusSelector  OutputSignals=TGB
  Bus Selector2 : BusSelector  OutputSignals=FBGG
  Bus Selector3 : BusSelector  OutputSignals=FBPB,MBPB
  Math Function : Math  Operator=transpose  SignedPower=on  SaturateOnIntegerOverflow=on
  Product : Product  Multiplication=Matrix(*)
  for_mom_bus : Outport  VectorParamsAs1DForOutWhenUnconnected=off
  wires:
  Bus Selector/1 -> Add/1  "<FBAB>"
  Bus Selector2/1 -> Product/2  "<FBGG>"
  Bus Selector1/1 -> Math Function/1  "<TGB>"
  Math Function/1 -> Product/1  "TBG"
  aero/1 -> Bus Selector/1
  Product/1 -> Add/2  "FBGB"
  prp/1 -> Bus Selector3/1
  motion_kin/1 -> Bus Selector1/1
  Add/1 -> Bus Creator/1  "FBTB"
  grav/1 -> Bus Selector2/1
  Add1/1 -> Bus Creator/2  "MBTB"
  Bus Selector/2 -> Add1/1  "<MBAB>"
  Bus Selector3/1 -> Add/3  "<FBPB>"
  Bus Creator/1 -> for_mom_bus/1  "for_mom_bus"
  Bus Selector3/2 -> Add1/2  "<MBPB>"

== system Mainframe/Non-linear Flight Dynamic Model/Subsystem1/GRM_Airframe/gravity ==
  env : Inport
  wab : Inport  Port=2
  Bus Creator3 : BusCreator  Inputs=1
  Bus Selector : BusSelector  OutputSignals=gBG,atm_bus.atm_stat_bus.hBE
  Bus Selector1 : BusSelector  OutputSignals=mB
  Product : Product
  launch_rail : Subsystem
  grav : Outport  VectorParamsAs1DForOutWhenUnconnected=off
  wires:
  launch_rail/1(gBG) -> Product/1
  Bus Selector/2 -> launch_rail/2(hBE)  "<hBE>"
  Bus Selector/1 -> launch_rail/1(gBG_c)  "<gBG>"
  Product/1 -> Bus Creator3/1  "FBGG"
  Bus Creator3/1 -> grav/1  "grav_bus"
  wab/1 -> Bus Selector1/1
  Bus Selector1/1 -> Product/2  "<mB>"
  env/1 -> Bus Selector/1

== system Mainframe/Non-linear Flight Dynamic Model/Subsystem1/GRM_Airframe/input ==
  siB_cmd : Inport
  Bus Creator2 : BusCreator  Inputs=1
  cmd_bus : Outport  VectorParamsAs1DForOutWhenUnconnected=off
  wires:
  siB_cmd/1 -> Bus Creator2/1
  Bus Creator2/1 -> cmd_bus/1  "cmd_bus"

== system Mainframe/Non-linear Flight Dynamic Model/Subsystem1/GRM_Airframe/motion_kinematics ==
  flight_dyn : Inport
  Bus Creator : BusCreator  Inputs=7
  Bus Selector : BusSelector  OutputSignals=lat,lon,qIB
  calc_motion_kinematics : Subsystem
  motion_kin : Outport  VectorParamsAs1DForOutWhenUnconnected=off
  wires:
  flight_dyn/1 -> Bus Selector/1
  Bus Creator/1 -> motion_kin/1  "motion_kin_bus"
  Bus Selector/1 -> calc_motion_kinematics/1(lat)  "<lat>"
  Bus Selector/2 -> calc_motion_kinematics/2(lon)  "<lon>"
  Bus Selector/3 -> calc_motion_kinematics/3(qIB)  "<qIB>"
  calc_motion_kinematics/1(wIEE) -> Bus Creator/1
  calc_motion_kinematics/2(TIE) -> Bus Creator/2
  calc_motion_kinematics/3(TEB) -> Bus Creator/3
  calc_motion_kinematics/4(TGB) -> Bus Creator/4
  calc_motion_kinematics/5(TEG) -> Bus Creator/5
  calc_motion_kinematics/6(wEGG) -> Bus Creator/6
  calc_motion_kinematics/7(TIB) -> Bus Creator/7

== system Mainframe/Non-linear Flight Dynamic Model/Subsystem1/GRM_Airframe/propulsion ==
  env_glbl : Inport
  wab : Inport  Port=2
  Bus Creator1 : BusCreator  Inputs=2
  prp_look_up : Subsystem
  prp_uncertainty : Subsystem
  prp : Outport  VectorParamsAs1DForOutWhenUnconnected=off
  wires:
  Bus Creator1/1 -> prp/1  "prp_bus"
  prp_look_up/1(FBPM) -> prp_uncertainty/1(FBPM)
  env_glbl/1 -> prp_look_up/1(env_glbl_bus)
  prp_uncertainty/2(MBPB) -> Bus Creator1/2
  prp_uncertainty/1(FBPB) -> Bus Creator1/1
  wab/1 -> prp_uncertainty/2(wab)

== system Mainframe/Non-linear Flight Dynamic Model/Subsystem1/GRM_Airframe/rb_eom ==
  mot_kin : Inport
  for_mom : Inport  Port=2
  wab : Inport  Port=3
  Bus Creator : BusCreator  Inputs=16
  calc_bus_flight_dyn_bus_entries : Subsystem
  eom_6dof : Subsystem
  flight_dyn : Outport  VectorParamsAs1DForOutWhenUnconnected=off
  wires:
  mot_kin/1 -> calc_bus_flight_dyn_bus_entries/1(mot_kin)
  calc_bus_flight_dyn_bus_entries/1(aBIB) -> Bus Creator/1
  calc_bus_flight_dyn_bus_entries/2(lon) -> Bus Creator/2
  calc_bus_flight_dyn_bus_entries/3(lat) -> Bus Creator/3
  calc_bus_flight_dyn_bus_entries/4(hBE) -> Bus Creator/4
  calc_bus_flight_dyn_bus_entries/5(vBII) -> Bus Creator/5
  calc_bus_flight_dyn_bus_entries/6(qIB) -> Bus Creator/6
  calc_bus_flight_dyn_bus_entries/7(wBIB) -> Bus Creator/7
  calc_bus_flight_dyn_bus_entries/8(d_wBIB) -> Bus Creator/8
  calc_bus_flight_dyn_bus_entries/9(d_vBII) -> Bus Creator/9
  Bus Creator/1 -> flight_dyn/1  "flight_dyn_bus"
  for_mom/1 -> eom_6dof/1(for_mom)
  wab/1 -> eom_6dof/2(wab)
  eom_6dof/1(eom) -> calc_bus_flight_dyn_bus_entries/2(eom)
  calc_bus_flight_dyn_bus_entries/10(pBII) -> Bus Creator/10
  calc_bus_flight_dyn_bus_entries/11(euIB) -> Bus Creator/11
  calc_bus_flight_dyn_bus_entries/12(vBIB) -> Bus Creator/12
  calc_bus_flight_dyn_bus_entries/13(qGB) -> Bus Creator/13
  calc_bus_flight_dyn_bus_entries/14(euGB) -> Bus Creator/14
  calc_bus_flight_dyn_bus_entries/15(euBG) -> Bus Creator/15
  calc_bus_flight_dyn_bus_entries/16(pBLG) -> Bus Creator/16

== system Mainframe/Non-linear Flight Dynamic Model/Subsystem1/GRM_Airframe/stream_flow ==
  flight_dyn : Inport
  motion_kin : Inport  Port=2
  env : Inport  Port=3
  Bus Selector1 : BusSelector  OutputSignals=atm_bus.atm_stat_bus.rho,atm_bus.atm_stat_bus.sos,atm_bus.atm_stat_bus.hBE
  Bus Selector2 : BusSelector  OutputSignals=vBII,pBII,wBIB
  Bus Selector3 : BusSelector  OutputSignals=TIB,wIEE,TIE
  calc_stream_flow : Subsystem
  str_flow : Outport  VectorParamsAs1DForOutWhenUnconnected=off
  wires:
  motion_kin/1 -> Bus Selector3/1
  flight_dyn/1 -> Bus Selector2/1
  env/1 -> Bus Selector1/1
  Bus Selector3/1 -> calc_stream_flow/1(TIB)  "<TIB>"
  Bus Selector3/2 -> calc_stream_flow/2(wIEE)  "<wIEE>"
  Bus Selector3/3 -> calc_stream_flow/3(TIE)  "<TIE>"
  Bus Selector2/1 -> calc_stream_flow/4(VBII)  "<vBII>"
  Bus Selector2/3 -> calc_stream_flow/6(wBIB)  "<wBIB>"
  Bus Selector1/1 -> calc_stream_flow/7(rho)  "<rho>"
  Bus Selector1/2 -> calc_stream_flow/8(sos)  "<sos>"
  Bus Selector1/3 -> calc_stream_flow/9(hBE)  "<hBE>"
  calc_stream_flow/1(str_flow) -> str_flow/1
  Bus Selector2/2 -> calc_stream_flow/5(pBII)  "<pBII>"

== system Mainframe/Non-linear Flight Dynamic Model/Subsystem1/GRM_Airframe/weight_and_balance ==
  env_glb : Inport
  Bus Creator1 : BusCreator  Inputs=3
  Bus Selector2 : BusSelector  OutputSignals=T_sim_glbl,T_sim_lnch
  Subtract : Sum  Inputs=+-
  center_of_gravity : Subsystem
  mass : Subsystem
  mass_uncertainty : Subsystem
  moi : Subsystem
  wab : Outport  VectorParamsAs1DForOutWhenUnconnected=off
  wires:
  Bus Selector2/2 -> Subtract/2  "<T_sim_lnch>"
  Bus Selector2/1 -> Subtract/1  "<T_sim_glbl>"
  env_glb/1 -> Bus Selector2/1
  Bus Creator1/1 -> wab/1  "wab_bus"
  center_of_gravity/1(pBPB) -> moi/1(pBPB), Bus Creator1/2
  moi/1(JBBB) -> Bus Creator1/3
  mass/2(mM) -> moi/2(mM), center_of_gravity/2(mM)
  mass_uncertainty/1(mB) -> center_of_gravity/1(mB), Bus Creator1/1
  mass/1(mB_c) -> mass_uncertainty/1(mB_c)
  Subtract/1 -> mass/1(sim_time_launch)

== system Mainframe/Servos/Real Servos/Reset Encoders/Triggered Subsystem ==
  In1 : Inport
  Enable : EnablePort
  Out1 : Outport
  wires:
  In1/1 -> Out1/1

== system Mainframe/Emulated FCC/Emulated Pixhawk/Autopilot/Phi_Control/Gain_Lookup ==
  V_mps : Inport
  h_m : Inport  Port=2
  1-D Lookup Table1 : Lookup_n-D  BreakpointsForDimension1=Autopilot.Ay.h_bkpts_m  BreakpointsForDimension2=Autopilot.Ay.V_bkpts_mps  Table=Autopilot.Ay.Kp_r_vec  ExtrapMethod=Clip  UseLastTableValue=on  InternalRulePriority=Speed  RndMeth=Simplest  InputSameDT=on
      settings: InputPortMap=u0,u1
      settings: AttributesFormatString=|
      | %<Table>
      | %<BreakpointsForDimension1>
      | %<BreakpointsForDimension2>
  1-D Lookup Table2 : Lookup_n-D  BreakpointsForDimension1=Autopilot.Ay.h_bkpts_m  BreakpointsForDimension2=Autopilot.Ay.V_bkpts_mps  Table=Autopilot.Ay.Kp_ay_vec  ExtrapMethod=Clip  UseLastTableValue=on  InternalRulePriority=Speed  RndMeth=Simplest  InputSameDT=on
      settings: InputPortMap=u0,u1
      settings: AttributesFormatString=|
      | %<Table>
      | %<BreakpointsForDimension1>
      | %<BreakpointsForDimension2>
  1-D Lookup Table3 : Lookup_n-D  BreakpointsForDimension1=Autopilot.Phi.h_bkpts_m  BreakpointsForDimension2=Autopilot.Phi.V_bkpts_mps  Table=Autopilot.Phi.Kp_p_vec  ExtrapMethod=Clip  UseLastTableValue=on  InternalRulePriority=Speed  RndMeth=Simplest  InputSameDT=on
      settings: InputPortMap=u0,u1
      settings: AttributesFormatString=|
      | %<Table>
      | %<BreakpointsForDimension1>
      | %<BreakpointsForDimension2>
  1-D Lookup Table4 : Lookup_n-D  BreakpointsForDimension1=Autopilot.Phi.h_bkpts_m  BreakpointsForDimension2=Autopilot.Phi.V_bkpts_mps  Table=Autopilot.Phi.Ki_phi_vec  ExtrapMethod=Clip  UseLastTableValue=on  InternalRulePriority=Speed  RndMeth=Simplest  InputSameDT=on
      settings: InputPortMap=u0,u1
      settings: AttributesFormatString=|
      | %<Table>
      | %<BreakpointsForDimension1>
      | %<BreakpointsForDimension2>
  1-D Lookup Table5 : Lookup_n-D  BreakpointsForDimension1=Autopilot.Phi.h_bkpts_m  BreakpointsForDimension2=Autopilot.Phi.V_bkpts_mps  Table=Autopilot.Phi.Kp_phi_vec  ExtrapMethod=Clip  UseLastTableValue=on  InternalRulePriority=Speed  RndMeth=Simplest  InputSameDT=on
      settings: InputPortMap=u0,u1
      settings: AttributesFormatString=|
      | %<Table>
      | %<BreakpointsForDimension1>
      | %<BreakpointsForDimension2>
  1-D Lookup Table6 : Lookup_n-D  BreakpointsForDimension1=Autopilot.Ay.h_bkpts_m  BreakpointsForDimension2=Autopilot.Ay.V_bkpts_mps  Table=Autopilot.Ay.Ki_ay_vec  ExtrapMethod=Clip  UseLastTableValue=on  InternalRulePriority=Speed  RndMeth=Simplest  InputSameDT=on
      settings: InputPortMap=u0,u1
      settings: AttributesFormatString=|
      | %<Table>
      | %<BreakpointsForDimension1>
      | %<BreakpointsForDimension2>
  Bus Creator1 : BusCreator  Inputs=6
  V_mps D{1..5} (5 alike) : InportShadow
  h_m D{1..5} (5 alike) : InportShadow  Port=2
  Gains : Outport
  wires:
  h_m/1 -> 1-D Lookup Table3/1
  Bus Creator1/1 -> Gains/1
  1-D Lookup Table5/1 -> Bus Creator1/3  "Kp_phi"
  1-D Lookup Table4/1 -> Bus Creator1/2  "Ki_phi"
  1-D Lookup Table3/1 -> Bus Creator1/1  "Kp_p"
  V_mps/1 -> 1-D Lookup Table3/2
  h_m D1/1 -> 1-D Lookup Table4/1
  V_mps D1/1 -> 1-D Lookup Table4/2
  h_m D2/1 -> 1-D Lookup Table5/1
  V_mps D2/1 -> 1-D Lookup Table5/2
  1-D Lookup Table2/1 -> Bus Creator1/6  "Kp_ay"
  1-D Lookup Table6/1 -> Bus Creator1/5  "Ki_ay"
  1-D Lookup Table1/1 -> Bus Creator1/4  "Kp_r"
  h_m D3/1 -> 1-D Lookup Table1/1
  V_mps D3/1 -> 1-D Lookup Table1/2
  h_m D4/1 -> 1-D Lookup Table6/1
  V_mps D4/1 -> 1-D Lookup Table6/2
  h_m D5/1 -> 1-D Lookup Table2/1
  V_mps D5/1 -> 1-D Lookup Table2/2

== system Mainframe/Flight Control Computer/FCC - Real or Emulated/Emulated FCC/Emulated Pixhawk/Autopilot ==
  Cmd : Inport
  IMU Data : Inport  Port=2
  INS Data : Inport  Port=3
  Bus Creator3 : BusCreator  Inputs=3
  Bus Selector : BusSelector  OutputSignals=phi_cmd
  Bus Selector1 : BusSelector  OutputSignals=gyro_x
  Bus Selector2 : BusSelector  OutputSignals=phi,z,p
  Calculate U : Subsystem
  Discrete Transfer Fcn : DiscreteTransferFcn  Numerator=[num_lpf_d]  Denominator=[den_lpf_d]
  Gain : Gain  Gain=-1
  Manual Switch : ManualSwitch
  Phi_Control : Subsystem
  Zero : Constant  Value=0  OutDataTypeStr=Inherit: Inherit via back propagation
  Attitude_Commands : Outport  VectorParamsAs1DForOutWhenUnconnected=off
  wires:
  Bus Selector1/1 -> Discrete Transfer Fcn/1  "<gyro_x>"
  IMU Data/1 -> Bus Selector1/1
  Calculate U/1(U) -> Phi_Control/5(V_mps)
  Zero/1 -> [Delta_Cmd_Psi], [Delta_Cmd_Theta]
  [Delta_Cmd_Phi] -> Bus Creator3/1  "Phi_Cmd_rad"
  [Delta_Cmd_Theta] -> Bus Creator3/2  "Theta_Cmd_rad"
  Bus Creator3/1 -> Attitude_Commands/1
  [Delta_Cmd_Psi] -> Bus Creator3/3  "Psi_Cmd_rad"
  Bus Selector/1 -> Phi_Control/1(phi_cmd_rad)  "<phi_cmd>"
  Cmd/1 -> Bus Selector/1
  INS Data/1 -> Calculate U/1(INS Data), Bus Selector2/1
  Bus Selector2/1 -> Phi_Control/2(phi_rad)  "<phi>"
  [rst] -> Phi_Control/4(Reset Integrators)
  Bus Selector2/2 -> Gain/1  "<z>"
  Gain/1 -> Phi_Control/6(h_m)
  Phi_Control/1(dela_cmd_rad) -> [Delta_Cmd_Phi]  "Phi_Cmd_rad"
  Discrete Transfer Fcn/1 -> Manual Switch/1
  Bus Selector2/3 -> Manual Switch/2  "<p>"
  Manual Switch/1 -> Phi_Control/3(p_rps)

== system Mainframe/Flight Control Computer/FCC - Real or Emulated/Emulated FCC/Emulated Pixhawk/Convert to Bus ==
  Input : Inport  OutDataTypeStr=single
  100Hz Reset : Subsystem
  Bus Creator1 : BusCreator  Inputs=6
  Bus Creator2 : BusCreator  Inputs=12
  Bus Creator3 : BusCreator  Inputs=1
  Demux : Demux  Outputs=23
  Heartbeat : Outport  InitialOutput=0
  Ext. Commands : Outport  Port=2  OutDataTypeStr=single  InitialOutput=0
  Enable INS Flag : Outport  Port=3  InitialOutput=0
  Missile States : Outport  Port=4  OutDataTypeStr=single  InitialOutput=[0 0 0 0 0 0 0 0 0 0]
  Real Gyros Flag : Outport  Port=5  InitialOutput=0
  Virtual IMU Data : Outport  Port=6  OutDataTypeStr=single  InitialOutput=[0 0 0 0 0 0 0 0 0 0]
  tag scope: FCC_Enable=global, rst=global
  wires:
  Demux/22 -> Bus Creator2/12  "psi"
  Demux/21 -> Bus Creator2/11  "theta"
  Demux/20 -> Bus Creator2/10  "phi"
  Demux/4 -> Real Gyros Flag/1  "Real Gyros Flag"
  Demux/5 -> Bus Creator2/1  "u"
  Demux/18 -> Bus Creator1/5  "gyro_y"
  Bus Creator1/1 -> Virtual IMU Data/1
  Demux/16 -> Bus Creator1/3  "acc_z"
  Demux/9 -> Bus Creator2/5  "y"
  Demux/14 -> Bus Creator1/1  "acc_x"
  Demux/17 -> Bus Creator1/4  "gyro_x"
  Demux/15 -> Bus Creator1/2  "acc_y"
  Demux/19 -> Bus Creator1/6  "gyro_z"
  Demux/12 -> Bus Creator2/8  "q"
  Demux/7 -> Bus Creator2/3  "w"
  Demux/10 -> Bus Creator2/6  "z"
  Demux/6 -> Bus Creator2/2  "v"
  Demux/11 -> Bus Creator2/7  "p"
  Demux/13 -> Bus Creator2/9  "r"
  Demux/23 -> Bus Creator3/1  "phi_cmd"
  Demux/8 -> Bus Creator2/4  "x"
  Bus Creator3/1 -> Ext. Commands/1
  Bus Creator2/1 -> Missile States/1
  Demux/1 -> [FCC_Enable]  "EnableFCC"
  Input/1 -> Demux/1
  Demux/2 -> 100Hz Reset/1(Heartbeat), Heartbeat/1  "Hearbeat"
  Demux/3 -> Enable INS Flag/1  "Enable INS Flag"
  100Hz Reset/1(RST) -> [rst]
